simulink model "Control_model"  (R2024b)
settings: Solver=FixedStepAuto  StartTime=0.0  StopTime=10.0  FixedStep=0.01  RelTol=1e-3
undefined symbols (not defined in the file or in its folder): TransmissionState
settings Model: Creator=nan  LastModifiedBy=nan

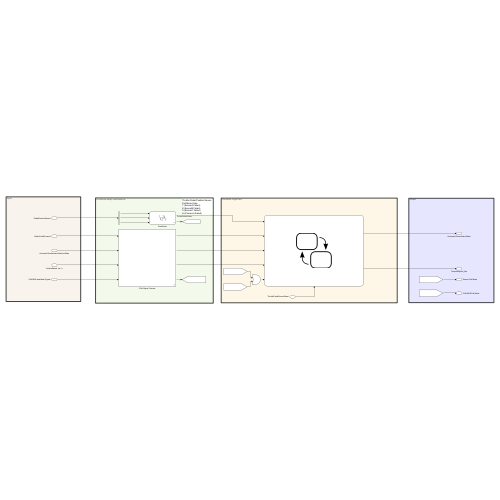
[thumbnail: Simulink's stored preview of the top-level diagram]
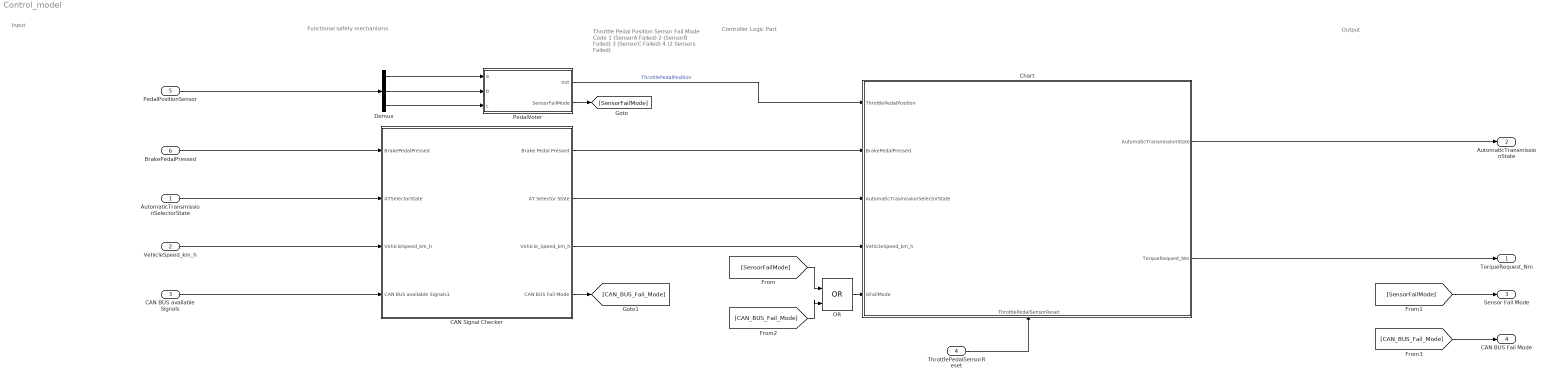
== system Control_model ==
  note: Input
  note: Functional safety mechanisms
  note: Throttle Pedal Position Sensor
      | Fail Mode Code
      | 1 (SensorA Failed)
      | 2 (SensorB Failed)
      | 3 (SensorC Failed)
      | 4 (2 Sensors Failed)
  note: Controller Logic Part
  note: Output
  AutomaticTransmissionSelectorState : Inport  OutDataTypeStr=Enum: TransmissionState
  VehicleSpeed_km_h : Inport  Port=2  OutDataTypeStr=single  Unit=km/h
  CAN BUS available Signals : Inport  Port=3  OutDataTypeStr=boolean  Unit=km/h
  ThrottlePedalSensorReset : Inport  Port=4  OutDataTypeStr=boolean  Unit=km/h
  PedalPositionSensor : Inport  Port=5
  BrakePedalPressed : Inport  Port=6  OutDataTypeStr=boolean
  CAN Signal Checker : Subsystem
  Chart : Stateflow chart  TreatAsAtomicUnit=on
      settings: PortSchema="{\"entries\":[{\"content\":{\"sides\":[{\"content\":{\"connectorIds\":[\"In2\",\"In1\",\"In3\",\"In4\",\"In6\"]},\"type\":\"ConnectorPlacement.EquallySpacedRectSide\",\"uuid\":\"7543a7ae-e0cf-4f10-8d78-a8beb38ca3e5\"},{\"content\":{\"connectorIds\":[\"Out1\",\"Out2\"],\"side\":\"RIGHT\"},\"type\":\"ConnectorPlacement.EquallySpacedRectSide\",\"uuid\":\"f0b83c8c-5e26-4afc-abc9-7bdae342d18a\"},{\"content\":{\"side\":\"TOP\"},\"type\":\"ConnectorPlacement.EquallySpacedRectSide\",\"uuid\":\"da051c3d-7aba-4992-b5fb-91af5925bb13\"},{\"content\":{\"connectorIds\":[\"In5\"],\"side\":\"BOTTOM\"},\"type\":\"ConnectorPlacement.EquallySpacedRectSide\",\"uuid\":\"e0d91eeb-09c2-4fcc-af74-b8f60f333922\"}]},\"type\":\"ConnectorPlacement.EquallySpacedConnector\",\"uuid\":\"6deea40b-4170-440f-abc0-6e54c3744eed\"}],\"packageUris\":[\"http://schema.mathworks.com/mf0/Connector/R2020b\"],\"version\":\"1.0\"}"
  Demux : Demux  Outputs=3
  OR : Logic  Operator=OR  IconShape=distinctive  AllPortsSameDT=off  OutDataTypeStr=boolean
  PedalVoter : Stateflow chart  TreatAsAtomicUnit=on
  TorqueRequest_Nm : Outport  OutDataTypeStr=single  Unit=N*m
  AutomaticTransmissionState : Outport  Port=2  OutDataTypeStr=Enum: TransmissionState
  Sensor Fail Mode : Outport  Port=3  OutDataTypeStr=int8
  CAN BUS Fail Mode : Outport  Port=4  OutDataTypeStr=int8
  wires:
  Chart/1(AutomaticTransmissionState) -> AutomaticTransmissionState/1
  Chart/2(TorqueRequest_Nm) -> TorqueRequest_Nm/1
  ThrottlePedalSensorReset/1 -> Chart/5(ThrottlePedalSensorReset)
  PedalPositionSensor/1 -> Demux/1
  Demux/1 -> PedalVoter/1(a)
  Demux/2 -> PedalVoter/2(b)
  Demux/3 -> PedalVoter/3(c)
  PedalVoter/2(SensorFailMode) -> [SensorFailMode]
  CAN BUS available Signals/1 -> CAN Signal Checker/4(CAN BUS available Signals1)
  VehicleSpeed_km_h/1 -> CAN Signal Checker/3(VehicleSpeed_km_h)
  AutomaticTransmissionSelectorState/1 -> CAN Signal Checker/2(ATSelectorState)
  BrakePedalPressed/1 -> CAN Signal Checker/1(BrakePedalPressed)
  PedalVoter/1(out) -> Chart/2(ThrottlePedalPosition)  "ThrottlePedalPosition"
  CAN Signal Checker/1(Brake Pedal Pressed) -> Chart/1(BrakePedalPressed)
  CAN Signal Checker/2(AT Selector State) -> Chart/3(AutomaticTrasmissionSelectorState)
  CAN Signal Checker/3(Vehicle_Speed_km_h) -> Chart/4(VehicleSpeed_km_h)
  OR/1 -> Chart/6(isFailMode)
  CAN Signal Checker/4(CAN BUS Fail Mode) -> [CAN_BUS_Fail_Mode]
  [SensorFailMode] -> OR/1
  [CAN_BUS_Fail_Mode] -> OR/2
  [SensorFailMode] -> Sensor Fail Mode/1
  [CAN_BUS_Fail_Mode] -> CAN BUS Fail Mode/1

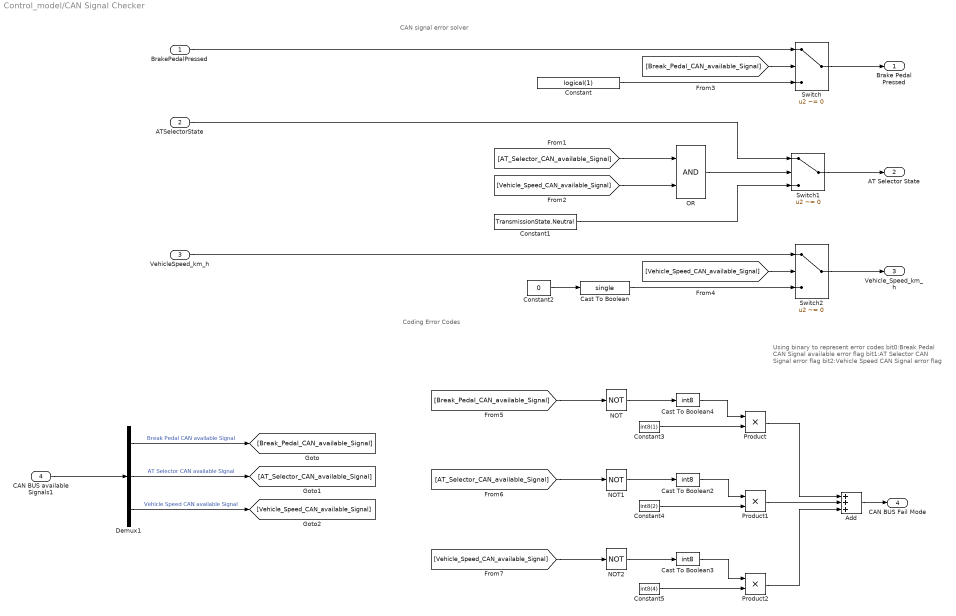
== system Control_model/CAN Signal Checker ==
  note: Coding Error Codes
  note: CAN signal error solver
  note: Using binary to represent error codes
      | bit0:Break Pedal CAN Signal available error flag
      | bit1:AT Selector CAN Signal error flag
      | bit2:Vehicle Speed CAN Signal error flag
  BrakePedalPressed : Inport
  ATSelectorState : Inport  Port=2
  VehicleSpeed_km_h : Inport  Port=3
  CAN BUS available Signals1 : Inport  Port=4
  Add : Sum  Inputs=+++
  Cast To Boolean : DataTypeConversion  OutDataTypeStr=single  SaturateOnIntegerOverflow=off  RndMeth=Floor
  Cast To Boolean2 : DataTypeConversion  OutDataTypeStr=int8  SaturateOnIntegerOverflow=off  RndMeth=Floor
  Cast To Boolean3 : DataTypeConversion  OutDataTypeStr=int8  SaturateOnIntegerOverflow=off  RndMeth=Floor
  Cast To Boolean4 : DataTypeConversion  OutDataTypeStr=int8  SaturateOnIntegerOverflow=off  RndMeth=Floor
  Constant : Constant  Value=logical(1)
  Constant1 : Constant  Value=TransmissionState.Neutral
  Constant2 : Constant  Value=0
  Constant3 : Constant  Value=int8(1)
  Constant4 : Constant  Value=int8(2)
  Constant5 : Constant  Value=int8(4)
  Demux1 : Demux  Outputs=3
  NOT : Logic  Operator=NOT  IconShape=distinctive  AllPortsSameDT=off  OutDataTypeStr=boolean
  NOT1 : Logic  Operator=NOT  IconShape=distinctive  AllPortsSameDT=off  OutDataTypeStr=boolean
  NOT2 : Logic  Operator=NOT  IconShape=distinctive  AllPortsSameDT=off  OutDataTypeStr=boolean
  OR : Logic  AllPortsSameDT=off  OutDataTypeStr=boolean
  Product : Product  OutDataTypeStr=int8
  Product1 : Product  OutDataTypeStr=int8
  Product2 : Product  OutDataTypeStr=int8
  Switch : Switch  Criteria=u2 ~= 0  SaturateOnIntegerOverflow=off  InputSameDT=off
  Switch1 : Switch  Criteria=u2 ~= 0  SaturateOnIntegerOverflow=off  InputSameDT=off
  Switch2 : Switch  Criteria=u2 ~= 0  SaturateOnIntegerOverflow=off  InputSameDT=off
  Brake Pedal Pressed : Outport
  AT Selector State : Outport  Port=2
  Vehicle_Speed_km_h : Outport  Port=3  OutDataTypeStr=single
  CAN BUS Fail Mode : Outport  Port=4
  wires:
  Demux1/3 -> [Vehicle_Speed_CAN_available_Signal]  "Vehicle Speed CAN available Signal"
  CAN BUS available Signals1/1 -> Demux1/1
  Demux1/1 -> [Break_Pedal_CAN_available_Signal]  "Break Pedal CAN available Signal"
  Demux1/2 -> [AT_Selector_CAN_available_Signal]  "AT Selector CAN available Signal"
  BrakePedalPressed/1 -> Switch/1
  Constant/1 -> Switch/3
  Switch/1 -> Brake Pedal Pressed/1
  [Break_Pedal_CAN_available_Signal] -> Switch/2
  [Vehicle_Speed_CAN_available_Signal] -> Switch2/2
  Constant2/1 -> Cast To Boolean/1
  Switch2/1 -> Vehicle_Speed_km_h/1
  VehicleSpeed_km_h/1 -> Switch2/1
  Cast To Boolean/1 -> Switch2/3
  ATSelectorState/1 -> Switch1/1
  OR/1 -> Switch1/2
  Constant1/1 -> Switch1/3
  [AT_Selector_CAN_available_Signal] -> OR/1
  [Vehicle_Speed_CAN_available_Signal] -> OR/2
  Switch1/1 -> AT Selector State/1
  [Vehicle_Speed_CAN_available_Signal] -> NOT2/1
  NOT/1 -> Cast To Boolean4/1
  [AT_Selector_CAN_available_Signal] -> NOT1/1
  Constant3/1 -> Product/2
  [Break_Pedal_CAN_available_Signal] -> NOT/1
  Cast To Boolean4/1 -> Product/1
  NOT2/1 -> Cast To Boolean3/1
  Constant5/1 -> Product2/2
  Cast To Boolean3/1 -> Product2/1
  NOT1/1 -> Cast To Boolean2/1
  Product1/1 -> Add/2
  Product2/1 -> Add/3
  Product/1 -> Add/1
  Constant4/1 -> Product1/2
  Cast To Boolean2/1 -> Product1/1
  Add/1 -> CAN BUS Fail Mode/1

== stateflow chart Control_model/PedalVoter ==
  state Normal
    du:
    abDiff = single(abs(a-b));
    acDiff = single(abs(a-c));
    bcDiff = single(abs(b-c));
    if   a<0 || a>1 || (abDiff>Tolerance && acDiff>Tolerance)  %%A failure
    out = (b+c)/2;
    SensorFailMode = 1;
    elseif b>1 || b<0 || abDiff>Tolerance  %%B failure
    out = (a+c)/2;
    SensorFailMode = 2;
    elseif c>1 || c<0 || acDiff>Tolerance %%C failure
    out = (a+b)/2;
    SensorFailMode = 3;
    else
    out = (a+b+c)/3;
    SensorFailMode = 0;
    end
  note: ?
  note: EmergencyMode Code
      | 1 (SensorA Failed)
      | 2 (SensorB Failed)
      | 3 (SensorC Failed)
      | 4 (2 Sensors Failed)
  state A_Failure
    en:
    out = (b+c)/2;
    du:
    bcDiff = abs(b-c);
    if bcDiff>Tolerance||b>1||b<0||c>1||c<0
    SensorFailMode = 4;
    out = 0;
    else
    out = (b+c)/2;
    end
  state B_Failure
    en:
    out = (a+c)/2;
    du:
    acDiff = abs(a-c);
    if acDiff>Tolerance||a>1||a<0||c>1||c<0
    SensorFailMode = 4;
    out = 0;
    else
    out = (a+c)/2;
    end
  state C_Failure
    en:
    out = (a+b)/2;
    du:
    abDiff = abs(a-b);
    if abDiff>Tolerance||b>1||b<0||a>1||a<0
    SensorFailMode = 4;
    out = 0;
    else
    out = (a+b)/2;
    end
  state NO_Trust
    en:
    out = 0;
  note: //Fail
  (default) -> Normal
  Normal -> C_Failure [order 2] : [SensorFailMode == 3]
  Normal -> A_Failure [order 1] : [SensorFailMode == 1]
  Normal -> B_Failure [order 3] : [SensorFailMode == 2]
  A_Failure -> NO_Trust : [SensorFailMode == 4]
  B_Failure -> NO_Trust : [SensorFailMode == 4]
  C_Failure -> NO_Trust : [SensorFailMode == 4]
  NO_Trust -> NO_Trust
  data: out output single; a input single; b input single; SensorFailMode output int8 =0; c input single; abDiff local single =0; acDiff local single =0; bcDiff local single =0; Tolerance local single =0.001

== stateflow chart Control_model/Chart ==
  state NoFailureDetected
    state Park
      en:
      AutomaticTransmissionState =TransmissionState.Park;
      du:
      TorqueRequest_Nm = 0;
    state Brake
      en:
      AutomaticTransmissionState =TransmissionState.Brake;
      state BrakeNormal
        state brakeAccle
          du:
          TorqueRequest_Nm = single(ThrottlePedalPosition-1/3)*1.5 * 960/12;
        state barkDecele
          du:
          TorqueRequest_Nm = -3*single(1/3-ThrottlePedalPosition) * 960/12;
        state brak0Velocity
          du:
          %Add a PI controller
          error = 0 - VehicleSpeed_km_h;
          sumError = sumError + error;
          TorqueRequest_Nm = error*30+sumError*2;
          ex:sumError = 0;
        (default) -> brakeAccle
        brakeAccle -> barkDecele : [ThrottlePedalPosition<=1/3]
        barkDecele -> brakeAccle [order 1] : [ThrottlePedalPosition>1/3]
        (junction 83) -> brakeAccle
        barkDecele -> brak0Velocity [order 2] : [VehicleSpeed_km_h <= 0.2]
        brak0Velocity -> (junction 83) : [ThrottlePedalPosition>1/3]
      state barkStop
        en:
        TorqueRequest_Nm = 0;
      barkStop -> BrakeNormal : [BrakePedalPressed ~=1]
      BrakeNormal -> barkStop : [BrakePedalPressed ==1]
      (default) -> barkStop
    state Drive
      en:
      AutomaticTransmissionState =TransmissionState.Drive;
      state normalDrive
        du:
        TorqueRequest_Nm = single(ThrottlePedalPosition) * 960/12;
      state driveStop
        du:
        TorqueRequest_Nm = 0;
      NoFailureDetected.Drive.normalDrive -> NoFailureDetected.Drive.driveStop : [BrakePedalPressed ==1]
      NoFailureDetected.Drive.driveStop -> NoFailureDetected.Drive.normalDrive : [BrakePedalPressed~=1]
      (default) -> NoFailureDetected.Drive.driveStop
    state Neutral
      en:
      AutomaticTransmissionState =TransmissionState.Neutral;
      du:
      TorqueRequest_Nm = 0;
    state Reverse
      en:
      AutomaticTransmissionState =TransmissionState.Reverse;
      state normalReverse
        du:
        TorqueRequest_Nm = -8*single(ThrottlePedalPosition) * 60/12;
      state reverseStop
        du:
        TorqueRequest_Nm = 0;
      NoFailureDetected.Reverse.normalReverse -> NoFailureDetected.Reverse.reverseStop : [BrakePedalPressed==1]
      NoFailureDetected.Reverse.reverseStop -> NoFailureDetected.Reverse.normalReverse : [BrakePedalPressed~=1]
      (default) -> NoFailureDetected.Reverse.reverseStop
    (default) -> NoFailureDetected.Park
    NoFailureDetected.Neutral -> Brake [order 4] : [VehicleSpeed_km_h<5&&VehicleSpeed_km_h>-5 &&...
        | BrakePedalPressed == 1 &&...
        | AutomaticTrasmissionSelectorState ==TransmissionState.Brake]
    NoFailureDetected.Park -> NoFailureDetected.Neutral : [BrakePedalPressed == 1 &&...
        | AutomaticTrasmissionSelectorState ~= TransmissionState.Park ]
    NoFailureDetected.Neutral -> NoFailureDetected.Park [order 1] : [VehicleSpeed_km_h<5 &&...
        | VehicleSpeed_km_h>-5 &&...
        | BrakePedalPressed == 1 &&...
        | AutomaticTrasmissionSelectorState == TransmissionState.Park ]
    NoFailureDetected.Drive -> NoFailureDetected.Neutral [order 1] : [AutomaticTrasmissionSelectorState ==TransmissionState.Neutral]
    Brake -> NoFailureDetected.Drive [order 1] : [AutomaticTrasmissionSelectorState ==TransmissionState.Drive]
    NoFailureDetected.Neutral -> NoFailureDetected.Reverse [order 2] : [VehicleSpeed_km_h<5 &&VehicleSpeed_km_h > -5&&...
        | BrakePedalPressed == 1 &&...
        | AutomaticTrasmissionSelectorState ==TransmissionState.Reverse]
    NoFailureDetected.Neutral -> NoFailureDetected.Drive [order 3] : [VehicleSpeed_km_h<5&&VehicleSpeed_km_h>-5 &&...
        | BrakePedalPressed == 1 &&...
        | AutomaticTrasmissionSelectorState ==TransmissionState.Drive]
    NoFailureDetected.Reverse -> NoFailureDetected.Neutral : [AutomaticTrasmissionSelectorState  ~= TransmissionState.Reverse]
    NoFailureDetected.Drive -> Brake [order 2] : [ThrottlePedalPosition>1/3 &&...
        | AutomaticTrasmissionSelectorState ==TransmissionState.Brake]
    Brake -> NoFailureDetected.Neutral [order 2] : [AutomaticTrasmissionSelectorState ==TransmissionState.Neutral]
  state LimpMode %When any sensor/CAN signal failure, enter this protect mode (with power constraints)
    state Park
      en:
      AutomaticTransmissionState = TransmissionState.Park;
      du:
      TorqueRequest_Nm = 0;
    state Drive
      en:
      AutomaticTransmissionState =TransmissionState.Drive;
      state normalDrive
        du:
        if VehicleSpeed_km_h < 20
        TorqueRequest_Nm = single(ThrottlePedalPosition) * 80 / 10;
        else
        TorqueRequest_Nm = 0;
        end
      state driveStop
        du:
        TorqueRequest_Nm = 0;
      LimpMode.Drive.normalDrive -> LimpMode.Drive.driveStop : [BrakePedalPressed ==1]
      LimpMode.Drive.driveStop -> LimpMode.Drive.normalDrive : [BrakePedalPressed~=1]
      (default) -> LimpMode.Drive.driveStop
    state Neutral
      en:
      AutomaticTransmissionState =TransmissionState.Neutral;
      du:
      TorqueRequest_Nm = 0;
    state Reverse
      en:
      AutomaticTransmissionState =TransmissionState.Reverse;
      state normalReverse
        du:
        TorqueRequest_Nm = -8*single(ThrottlePedalPosition) * 60/12/10;
      state reverseStop
        du:
        TorqueRequest_Nm = 0;
      LimpMode.Reverse.normalReverse -> LimpMode.Reverse.reverseStop : [BrakePedalPressed == 1]
      LimpMode.Reverse.reverseStop -> LimpMode.Reverse.normalReverse : [BrakePedalPressed ~= 1]
      (default) -> LimpMode.Reverse.reverseStop
    (default) -> (junction 134)
    (junction 134) -> (junction 127) [order 4] : [lastTimeMode == TransmissionState.Reverse]
    (junction 134) -> LimpMode.Park [order 5]
    (junction 134) -> LimpMode.Drive [order 3] : [lastTimeMode == TransmissionState.Brake]
    (junction 134) -> LimpMode.Neutral [order 1] : [lastTimeMode == TransmissionState.Neutral]
    (junction 134) -> LimpMode.Drive [order 2] : [lastTimeMode == TransmissionState.Drive]
    (junction 127) -> LimpMode.Reverse
    LimpMode.Park -> LimpMode.Neutral : [BrakePedalPressed == 1 &&...
        | AutomaticTrasmissionSelectorState ~= TransmissionState.Park ]
    LimpMode.Neutral -> LimpMode.Park [order 1] : [VehicleSpeed_km_h<5 &&...
        | VehicleSpeed_km_h>-5 &&...
        | BrakePedalPressed == 1 &&...
        | AutomaticTrasmissionSelectorState == TransmissionState.Park ]
    LimpMode.Drive -> LimpMode.Neutral : [AutomaticTrasmissionSelectorState == TransmissionState.Neutral]
    LimpMode.Neutral -> LimpMode.Reverse [order 2] : [VehicleSpeed_km_h < 5 &&...
        |  VehicleSpeed_km_h > -5 &&...
        | BrakePedalPressed == 1 &&...
        | AutomaticTrasmissionSelectorState == TransmissionState.Reverse]
    LimpMode.Neutral -> LimpMode.Drive [order 3] : [VehicleSpeed_km_h> -5 &&...
        |  VehicleSpeed_km_h > -5 &&...
        | BrakePedalPressed == 1 &&...
        | (AutomaticTrasmissionSelectorState ==TransmissionState.Drive ||...
        | AutomaticTrasmissionSelectorState ==TransmissionState.Brake) ]
    LimpMode.Reverse -> LimpMode.Neutral : [AutomaticTrasmissionSelectorState  ~= TransmissionState.Reverse]
  (default) -> NoFailureDetected
  NoFailureDetected -> LimpMode %When any sensor/CAN signal failure, enter this protect mode (with power constraints) : [isFailMode ~= 0]
      | {lastTimeMode = AutomaticTransmissionState;}
  LimpMode %When any sensor/CAN signal failure, enter this protect mode (with power constraints) -> NoFailureDetected : [ThrottlePedalSensorReset == true && ...
      |  isFailMode == false]
  data: AutomaticTransmissionState output; BrakePedalPressed input; ThrottlePedalPosition input; AutomaticTrasmissionSelectorState input; VehicleSpeed_km_h input; TorqueRequest_Nm output single; sumError local single =0; error local; ThrottlePedalSensorReset input; isFailMode input; lastTimeMode local
